simulink model "AC_Feeder"  (R2016b)
settings: Solver=ode1  StartTime=0.0  StopTime=Tsim  FixedStep=Ts  MaxStep=Tsw/20  RelTol=1e-4  EnableMultiTasking=on
values from neighbouring files (symbols this model uses):
  C = 100e-6    (= 0.0001)    [AC_Feeder_Control_Param.m]    (also in AC_Feeder_Control_Param_02-CORPGYEGTI03-P.m; AC_Feeder_Control_Param_02.m; AC_Feeder_Param.m)
  K_pll = dcgain(Gc_pll/tf([1 -Z_pll],[1 -P_pll 0]))    [AC_Feeder_Control_Param.m]    (also in AC_Feeder_Control_Param_02-CORPGYEGTI03-P.m; AC_Feeder_Control_Param_02.m; AC_Feeder_Param.m; gcpll.m)
  Ll = 10e-3    (= 0.01)    [AC_Feeder_Control_Param.m]    (also in AC_Feeder_Control_Param_02-CORPGYEGTI03-P.m; AC_Feeder_Control_Param_02.m; AC_Feeder_Param.m)
  P_pll = res(2)    [AC_Feeder_Control_Param.m]    (also in AC_Feeder_Control_Param_02-CORPGYEGTI03-P.m; AC_Feeder_Control_Param_02.m; AC_Feeder_Param.m = ans(2); gcpll.m = res(1))
  R = 10    [AC_Feeder_Control_Param.m]    (also in AC_Feeder_Control_Param_02-CORPGYEGTI03-P.m; AC_Feeder_Control_Param_02.m; AC_Feeder_Param.m)
  Rl = 0.1    [AC_Feeder_Control_Param.m]    (also in AC_Feeder_Control_Param_02-CORPGYEGTI03-P.m; AC_Feeder_Control_Param_02.m; AC_Feeder_Param.m)
  Ts = 50e-6    (= 5e-05)    [AC_Feeder_Control_Param.m]    (also in AC_Feeder_Control_Param_02-CORPGYEGTI03-P.m; AC_Feeder_Control_Param_02.m; AC_Feeder_Param.m; Feeder_Param.m = 0.0001)
  Tsim = 1    [AC_Feeder_Control_Param.m]    (also in AC_Feeder_Control_Param_02-CORPGYEGTI03-P.m; AC_Feeder_Control_Param_02.m; AC_Feeder_Param.m)
  VLNpk = VLNrms*sqrt(2)    [AC_Feeder_Control_Param.m]    (also in AC_Feeder_Control_Param_02-CORPGYEGTI03-P.m; AC_Feeder_Control_Param_02.m; AC_Feeder_Param.m = VLLrms*sqrt(2/3))
  w1 = 2*pi*f1    (= 376.991118431)    [AC_Feeder_Control_Param.m]    (also in AC_Feeder_Control_Param_02-CORPGYEGTI03-P.m; AC_Feeder_Control_Param_02.m; AC_Feeder_Param.m)
  Z_pll = zero(Gc_pll)    [AC_Feeder_Control_Param.m]    (also in AC_Feeder_Control_Param_02-CORPGYEGTI03-P.m; AC_Feeder_Control_Param_02.m; AC_Feeder_Param.m; gcpll.m)
undefined symbols (not defined in the file or in its folder): DiscIntNeverNeededParam
libraries: powerlib x22, simulink x2
settings Model: Creator=daniel  LastModifiedBy=sixifo
settings DataIOCC: LimitDataPoints=on  SaveFormat=Array  SignalLoggingSaveFormat=ModelDataLogs
settings OptimizationCC: ExpressionDepthLimit=2147483647  InitFltsAndDblsToZero=on  LifeSpan=inf
settings DebuggingCC: UnderspecifiedInitializationDetection=Classic  MergeDetectMultiDrivingBlocksExec=none  SolverPrmCheckMsg=warning  FcnCallInpInsideContextMsg=warning  UnconnectedInputMsg=none  UnconnectedOutputMsg=none  UnconnectedLineMsg=none  StateNameClashWarn=warning  SFUnexpectedBacktrackingDiag=warning  SFNoUnconditionalDefaultTransitionDiag=warning  SFExecutionAtInitializationDiag=none
settings HardwareCC: ProdBitPerPointer=32  ProdBitPerSizeT=32  ProdBitPerPtrDiffT=32  ProdLargestAtomicFloat=None  ProdIntDivRoundTo=Undefined  ProdEndianess=Unspecified  ProdWordSize=32  ProdHWDeviceType=32-bit Generic
settings ModelReferenceCC: PropagateSignalLabelsOutOfModel=off
settings GRTTargetCC: TargetLangStandard=C89/C90 (ANSI)  CombineOutputUpdateFcns=off  GRTInterface=on
settings ConfigComp: CovMetricSettings=dw  CovHtmlReporting=on  CovSaveCumulativeToWorkspaceVar=on  CovSaveSingleToWorkspaceVar=on  CovExternalEMLEnable=off

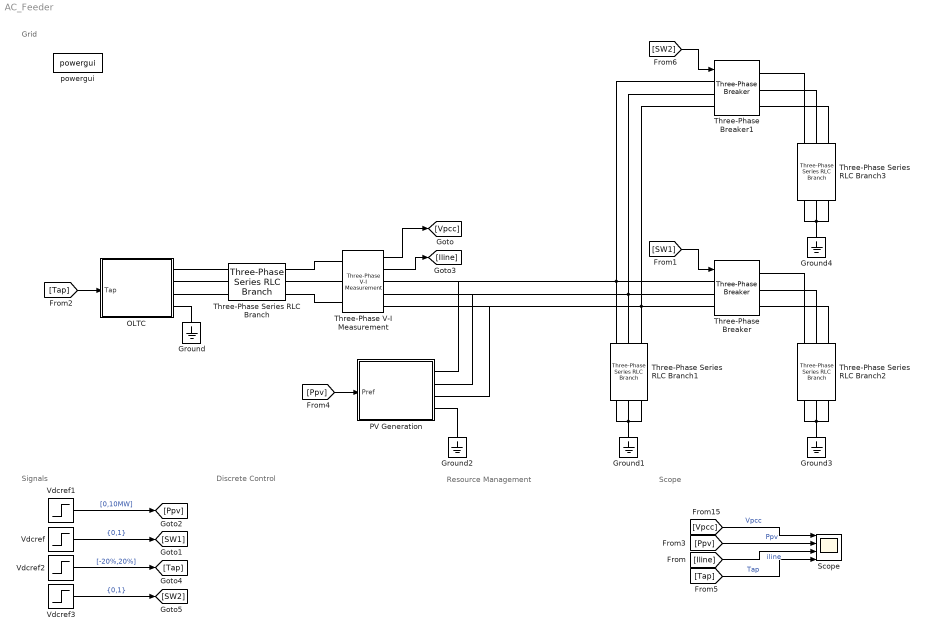
== system AC_Feeder ==
  note: Resource Management
  note: Signals
  note: Discrete Control
  note: Scope
  note: Grid
  Ground{,1..4} (5 alike) : powerlib/Elements/Ground  LConnTagsString=a
  OLTC : Subsystem
  PV Generation : Subsystem
  Scope : Scope  NumInputPorts=4
  Three-Phase Series RLC Branch : powerlib/Elements/Three-Phase Series RLC Branch  LConnTagsString=A|B|C  RConnTagsString=A|B|C  BranchType=RL  Resistance=Rl  Inductance=Ll  Capacitance=1e-6  Measurements=None
  Three-Phase Series RLC Branch1 : powerlib/Elements/Three-Phase Series RLC Branch  LConnTagsString=A|B|C  RConnTagsString=A|B|C  BranchType=R  Resistance=R  Inductance=Ll  Capacitance=1e-6  Measurements=None
  Three-Phase Series RLC Branch2 : powerlib/Elements/Three-Phase Series RLC Branch  LConnTagsString=A|B|C  RConnTagsString=A|B|C  BranchType=R  Resistance=R  Inductance=Ll  Capacitance=1e-6  Measurements=None
  Three-Phase Series RLC Branch3 : powerlib/Elements/Three-Phase Series RLC Branch  LConnTagsString=A|B|C  RConnTagsString=A|B|C  BranchType=C  Resistance=R  Inductance=Ll  Capacitance=C  Measurements=None
  Three-Phase V-I Measurement : powerlib/Measurements/Three-Phase V-I Measurement  VoltageMeasurement=phase-to-ground  SetLabelV=off  LabelV=Vabc  Vpu=off  VpuLL=off  CurrentMeasurement=yes  SetLabelI=off  LabelI=Iabc  Ipu=off  Pbase=100e6  Vbase=500e3  OutputType=Complex  PhasorSimulation=off  PSBequivalent=0
  Three-Phase Breaker : powerlib/Elements/Three-Phase Breaker  InitialState=open  SwitchA=on  SwitchB=on  SwitchC=on  SwitchTimes="[1/60  5/60]"  External=on  BreakerResistance=Ron  SnubberResistance=Rsnubber  SnubberCapacitance=inf  Measurements=None
  Three-Phase Breaker1 : powerlib/Elements/Three-Phase Breaker  InitialState=open  SwitchA=on  SwitchB=on  SwitchC=on  SwitchTimes="[1/60  5/60]"  External=on  BreakerResistance=Ron  SnubberResistance=Rsnubber  SnubberCapacitance=inf  Measurements=None
  Vdcref : Step  Time=Tsim*0.4  SampleTime=0
  Vdcref1 : Step  Time=Tsim*0.20  After=10e6  SampleTime=0
  Vdcref2 : Step  Time=Tsim*0.60  After=10  SampleTime=0
  Vdcref3 : Step  Time=Tsim*0.80  SampleTime=0
  powergui : powerlib/powergui  SimulationMode=Discrete  SolverType=Tustin/Backward Euler (TBE)  SampleTime=50e-6  frequency=60  SPID=off  DisableSnubberDevices=off  DisableRonSwitches=off  DisableVfSwitches=off  SwTol=0  DisplayEquations=off  Interpol=off  ExternalGateDelay=off  methode=off  Ts=0  FunctionMessages=off  echomessages=off  HookPort=off  EnableUseOfTLC=off  x0status=blocks  frequencyindice=0  Pbase=100e6  ErrMax=1e-4  Iterations=50  UnitsV=kV  UnitsW=MW  buscounter=0  RestoreLinks=warning  ResistiveCurrentMeasurement=off  Frange=[0:2:500]  Ylog=off  Xlog=on  ShowGrid=off  save=off  variable=ZData  structure=IL  ZoomFFT=off  StartTime=0  cycles=1  DisplayStyle=1  fundamental=1e4  FreqAxis=off  MaxFrequency=10000  frequencyindicesteady=1  RmsSteady=1  display=off
  wires:
  Vdcref/1 -> [SW1]  "{0,1}"
  [Ppv] -> Scope/2  "Ppv"
  [Tap] -> Scope/4  "Tap"
  [Vpcc] -> Scope/1  "Vpcc"
  [Ppv] -> PV Generation/1(Pref)
  [Iline] -> Scope/3  "iline"
  Vdcref1/1 -> [Ppv]  "[0,10MW]"
  [SW1] -> Three-Phase Breaker/1
  Three-Phase V-I Measurement/1 -> [Vpcc]
  Three-Phase V-I Measurement/2 -> [Iline]
  Vdcref2/1 -> [Tap]  "[-20%,20%]"
  [Tap] -> OLTC/1(Tap)
  Vdcref3/1 -> [SW2]  "{0,1}"
  [SW2] -> Three-Phase Breaker1/1
  connections:
  Ground1/LConn1 -- Three-Phase Series RLC Branch1/RConn3 -- Three-Phase Series RLC Branch1/RConn1 -- Three-Phase Series RLC Branch1/RConn2
  OLTC/RConn1 -- Three-Phase Series RLC Branch/LConn1
  OLTC/RConn2 -- Three-Phase Series RLC Branch/LConn2
  OLTC/RConn3 -- Three-Phase Series RLC Branch/LConn3
  Three-Phase V-I Measurement/RConn1 -- PV Generation/RConn1 -- Three-Phase Breaker1/LConn1 -- Three-Phase Breaker/LConn1 -- Three-Phase Series RLC Branch1/LConn1
  Three-Phase V-I Measurement/RConn2 -- PV Generation/RConn2 -- Three-Phase Breaker1/LConn2 -- Three-Phase Breaker/LConn2 -- Three-Phase Series RLC Branch1/LConn2
  Three-Phase V-I Measurement/RConn3 -- PV Generation/RConn3 -- Three-Phase Breaker1/LConn3 -- Three-Phase Breaker/LConn3 -- Three-Phase Series RLC Branch1/LConn3
  PV Generation/RConn4 -- Ground2/LConn1
  Ground3/LConn1 -- Three-Phase Series RLC Branch2/RConn3 -- Three-Phase Series RLC Branch2/RConn1 -- Three-Phase Series RLC Branch2/RConn2
  Three-Phase Breaker/RConn3 -- Three-Phase Series RLC Branch2/LConn3
  Three-Phase Breaker/RConn2 -- Three-Phase Series RLC Branch2/LConn2
  Three-Phase Breaker/RConn1 -- Three-Phase Series RLC Branch2/LConn1
  Three-Phase Series RLC Branch/RConn2 -- Three-Phase V-I Measurement/LConn2
  Three-Phase Series RLC Branch/RConn1 -- Three-Phase V-I Measurement/LConn1
  Three-Phase Series RLC Branch/RConn3 -- Three-Phase V-I Measurement/LConn3
  OLTC/RConn4 -- Ground/LConn1
  Ground4/LConn1 -- Three-Phase Series RLC Branch3/RConn3 -- Three-Phase Series RLC Branch3/RConn1 -- Three-Phase Series RLC Branch3/RConn2
  Three-Phase Series RLC Branch3/LConn2 -- Three-Phase Breaker1/RConn2
  Three-Phase Breaker1/RConn3 -- Three-Phase Series RLC Branch3/LConn3
  Three-Phase Breaker1/RConn1 -- Three-Phase Series RLC Branch3/LConn1

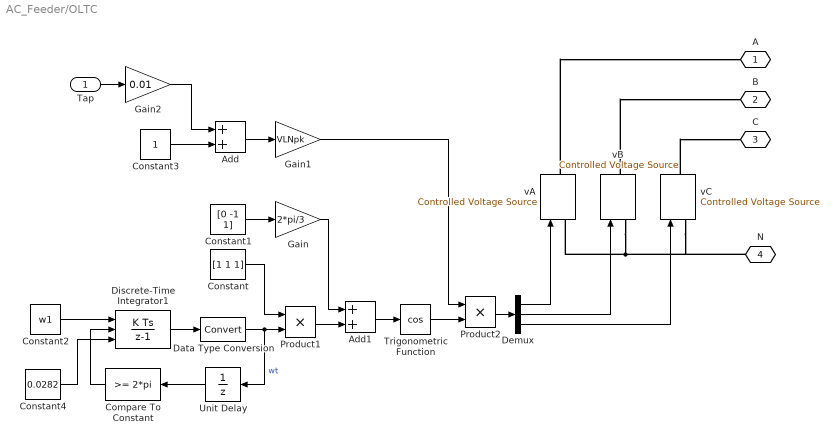
== system AC_Feeder/OLTC ==
  Tap : Inport
  Add : Sum
  Add1 : Sum
  Compare To Constant : simulink/Logic and Bit Operations/Compare To Constant  relop=>=  const=2*pi  OutDataTypeStr=boolean
  Constant : Constant  Value=[1 1 1]
  Constant1 : Constant  Value=[0 -1 1]
  Constant2 : Constant  Value=w1
  Constant3 : Constant
  Constant4 : Constant  Value=0.0282
  Data Type Conversion : DataTypeConversion
  Demux : Demux  Outputs=3
  Discrete-Time Integrator1 : DiscreteIntegrator  gainval=1  ExternalReset=rising  InitialConditionSource=external  SampleTime=Ts  UpperSaturationLimit=0.5*pi  LowerSaturationLimit=0.0001  ICPrevOutput=DiscIntNeverNeededParam  ICPrevScaledInput=DiscIntNeverNeededParam
  Gain : Gain  Gain=2*pi/3
  Gain1 : Gain  Gain=VLNpk
  Gain2 : Gain  Gain=0.01
  Product1 : Product
  Product2 : Product
  Trigonometric Function : Trigonometry  Operator=cos
  Unit Delay : UnitDelay  SampleTime=-1
  vA : powerlib/Electrical Sources/Controlled Voltage Source  Initialize=on  Source_Type=AC  Amplitude=0  Phase=0  Frequency=0  Measurements=None
  vB : powerlib/Electrical Sources/Controlled Voltage Source  Initialize=on  Source_Type=AC  Amplitude=0  Phase=0  Frequency=0  Measurements=None
  vC : powerlib/Electrical Sources/Controlled Voltage Source  Initialize=on  Source_Type=AC  Amplitude=0  Phase=0  Frequency=0  Measurements=None
  A : PMIOPort  Port=1  Side=Right
  B : PMIOPort  Port=2  Side=Right
  C : PMIOPort  Port=3  Side=Right
  N : PMIOPort  Port=4  Side=Right
  wires:
  Demux/1 -> vA/1
  Demux/2 -> vB/1
  Demux/3 -> vC/1
  Product1/1 -> Add1/2
  Constant1/1 -> Gain/1
  Add1/1 -> Trigonometric Function/1
  Constant/1 -> Product1/1
  Gain/1 -> Add1/1
  Trigonometric Function/1 -> Product2/2
  Product2/1 -> Demux/1
  Add/1 -> Gain1/1
  Constant3/1 -> Add/2
  Gain1/1 -> Product2/1
  Gain2/1 -> Add/1
  Tap/1 -> Gain2/1
  Data Type Conversion/1 -> Unit Delay/1, Product1/2  "wt"
  Unit Delay/1 -> Compare To Constant/1
  Discrete-Time Integrator1/1 -> Data Type Conversion/1
  Compare To Constant/1 -> Discrete-Time Integrator1/2
  Constant4/1 -> Discrete-Time Integrator1/3
  Constant2/1 -> Discrete-Time Integrator1/1
  connections:
  vB/LConn1 -- N/RConn1 -- vC/LConn1 -- vA/LConn1
  vA/RConn1 -- A/RConn1
  vB/RConn1 -- B/RConn1
  vC/RConn1 -- C/RConn1

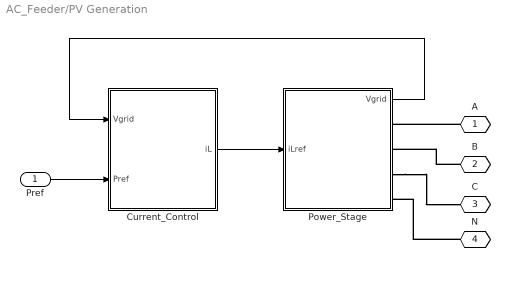
== system AC_Feeder/PV Generation ==
  Pref : Inport
  Current_Control : Subsystem
  Power_Stage : Subsystem
  A : PMIOPort  Port=1  Side=Right
  B : PMIOPort  Port=2  Side=Right
  C : PMIOPort  Port=3  Side=Right
  N : PMIOPort  Port=4  Side=Right
  wires:
  Pref/1 -> Current_Control/2(Pref)
  Power_Stage/1(Vgrid) -> Current_Control/1(Vgrid)
  Current_Control/1(iL) -> Power_Stage/1(iLref)
  connections:
  A/RConn1 -- Power_Stage/RConn1
  B/RConn1 -- Power_Stage/RConn2
  Power_Stage/RConn3 -- C/RConn1
  N/RConn1 -- Power_Stage/RConn4

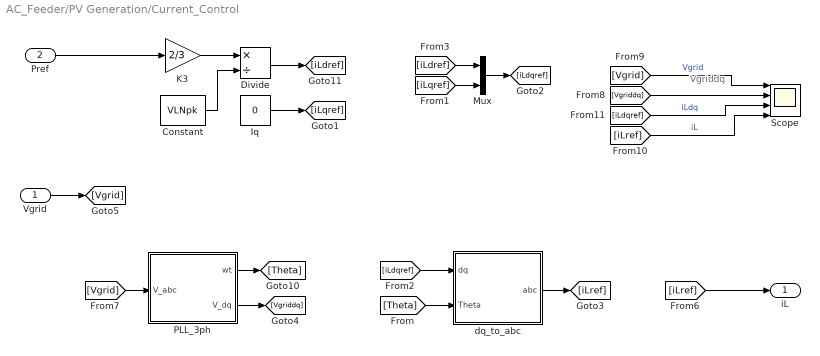
== system AC_Feeder/PV Generation/Current_Control ==
  note: Vgriddq
  Vgrid : Inport
  Pref : Inport  Port=2
  Constant : Constant  Value=VLNpk
  Divide : Product  Inputs=*/
  Iq : Constant  Value=0
  K3 : Gain  Gain=2/3
  Mux : Mux  Inputs=2
  PLL_3ph : Subsystem
  Scope : Scope  NumInputPorts=4
  dq_to_abc : Subsystem
  iL : Outport
  wires:
  [iLdref] -> Mux/1
  K3/1 -> Divide/1
  Pref/1 -> K3/1
  Constant/1 -> Divide/2
  Divide/1 -> [iLdref]
  [iLqref] -> Mux/2
  [Vgrid] -> PLL_3ph/1(V_abc)
  PLL_3ph/2(V_dq) -> [Vgriddq]
  PLL_3ph/1(wt) -> [Theta]
  Vgrid/1 -> [Vgrid]
  Iq/1 -> [iLqref]
  Mux/1 -> [iLdqref]
  [Theta] -> dq_to_abc/2(Theta)
  [iLdqref] -> dq_to_abc/1(dq)
  dq_to_abc/1(abc) -> [iLref]
  [iLref] -> iL/1
  [Vgriddq] -> Scope/2
  [Vgrid] -> Scope/1  "Vgrid"
  [iLdqref] -> Scope/3  "iLdq"
  [iLref] -> Scope/4  "iL"

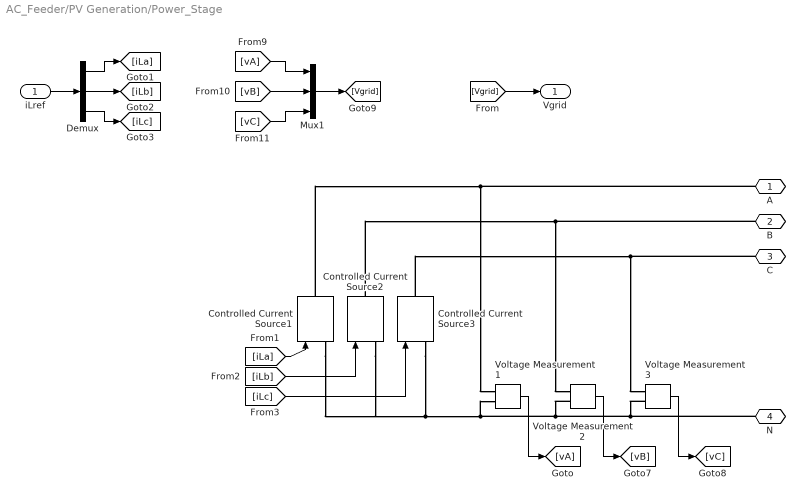
== system AC_Feeder/PV Generation/Power_Stage ==
  iLref : Inport
  Controlled Current Source1 : powerlib/Electrical Sources/Controlled Current Source  Initialize=on  Source_Type=AC  Amplitude=0  Phase=0  Frequency=0  Measurements=None
  Controlled Current Source2 : powerlib/Electrical Sources/Controlled Current Source  Initialize=on  Source_Type=AC  Amplitude=0  Phase=0  Frequency=0  Measurements=None
  Controlled Current Source3 : powerlib/Electrical Sources/Controlled Current Source  Initialize=on  Source_Type=AC  Amplitude=0  Phase=0  Frequency=0  Measurements=None
  Demux : Demux  Outputs=3
  Mux1 : Mux  Inputs=3
  Voltage Measurement 1 : powerlib/Measurements/Voltage Measurement  PhasorSimulation=off  OutputType=Complex  PSBequivalent=0
  Voltage Measurement 2 : powerlib/Measurements/Voltage Measurement  PhasorSimulation=off  OutputType=Complex  PSBequivalent=0
  Voltage Measurement 3 : powerlib/Measurements/Voltage Measurement  PhasorSimulation=off  OutputType=Complex  PSBequivalent=0
  A : PMIOPort  Port=1  Side=Right
  B : PMIOPort  Port=2  Side=Right
  C : PMIOPort  Port=3  Side=Right
  N : PMIOPort  Port=4  Side=Right
  Vgrid : Outport
  wires:
  Voltage Measurement 3/1 -> [vC]
  Voltage Measurement 2/1 -> [vB]
  Voltage Measurement 1/1 -> [vA]
  Mux1/1 -> [Vgrid]
  [vC] -> Mux1/3
  [vA] -> Mux1/1
  [vB] -> Mux1/2
  [Vgrid] -> Vgrid/1
  iLref/1 -> Demux/1
  Demux/1 -> [iLa]
  Demux/2 -> [iLb]
  Demux/3 -> [iLc]
  [iLa] -> Controlled Current Source1/1
  [iLb] -> Controlled Current Source2/1
  [iLc] -> Controlled Current Source3/1
  connections:
  Voltage Measurement 3/LConn2 -- N/RConn1 -- Controlled Current Source1/LConn1 -- Controlled Current Source2/LConn1 -- Controlled Current Source3/LConn1 -- Voltage Measurement 1/LConn2 -- Voltage Measurement 2/LConn2
  C/RConn1 -- Controlled Current Source3/RConn1 -- Voltage Measurement 3/LConn1
  B/RConn1 -- Controlled Current Source2/RConn1 -- Voltage Measurement 2/LConn1
  A/RConn1 -- Controlled Current Source1/RConn1 -- Voltage Measurement 1/LConn1

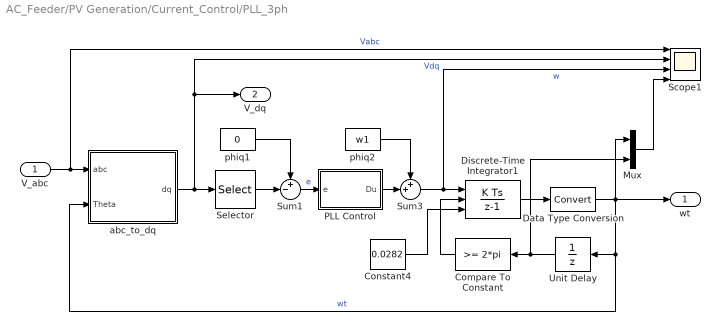
== system AC_Feeder/PV Generation/Current_Control/PLL_3ph ==
  V_abc : Inport
  Compare To Constant : simulink/Logic and Bit Operations/Compare To Constant  relop=>=  const=2*pi  OutDataTypeStr=boolean
  Constant4 : Constant  Value=0.0282
  Data Type Conversion : DataTypeConversion
  Discrete-Time Integrator1 : DiscreteIntegrator  gainval=1  ExternalReset=rising  InitialConditionSource=external  SampleTime=Ts  UpperSaturationLimit=0.5*pi  LowerSaturationLimit=0.0001  ICPrevOutput=DiscIntNeverNeededParam  ICPrevScaledInput=DiscIntNeverNeededParam
  Mux : Mux  Inputs=2
  PLL Control : Subsystem
  Scope1 : Scope  NumInputPorts=4
  Selector : Selector  InputPortWidth=2  IndexOptions=Index vector (dialog)  Indices=[2]  OutputSizes=1
  Sum1 : Sum  Inputs=+-|  SaturateOnIntegerOverflow=on
  Sum3 : Sum  Inputs=++|  SaturateOnIntegerOverflow=on
  Unit Delay : UnitDelay  SampleTime=-1
  abc_to_dq : Subsystem
  phiq1 : Constant  Value=0  OutDataTypeStr=single
  phiq2 : Constant  Value=w1  OutDataTypeStr=single
  wt : Outport
  V_dq : Outport  Port=2
  wires:
  Sum3/1 -> Scope1/3, Discrete-Time Integrator1/1  "w"
  phiq2/1 -> Sum3/1
  V_abc/1 -> abc_to_dq/1(abc), Scope1/1  "Vabc"
  Discrete-Time Integrator1/1 -> Data Type Conversion/1
  Compare To Constant/1 -> Discrete-Time Integrator1/2
  Constant4/1 -> Discrete-Time Integrator1/3
  PLL Control/1(Du) -> Sum3/2
  abc_to_dq/1(dq) -> Selector/1, V_dq/1, Scope1/2  "Vdq"
  Sum1/1 -> PLL Control/1(e)  "e"
  phiq1/1 -> Sum1/1
  Selector/1 -> Sum1/2
  Data Type Conversion/1 -> Mux/1, Unit Delay/1, abc_to_dq/2(Theta), wt/1  "wt"
  Unit Delay/1 -> Mux/2, Compare To Constant/1
  Mux/1 -> Scope1/4

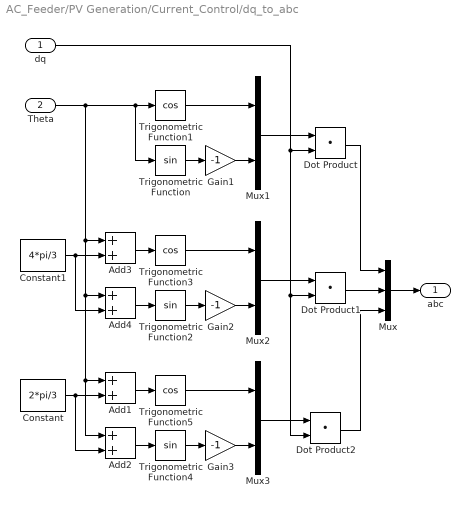
== system AC_Feeder/PV Generation/Current_Control/dq_to_abc ==
  dq : Inport
  Theta : Inport  Port=2
  Add{1..4} (4 alike) : Sum
  Constant : Constant  Value=2*pi/3
  Constant1 : Constant  Value=4*pi/3
  Dot Product : DotProduct  InputSameDT=on  OutDataTypeStr=Inherit: Inherit via internal rule
  Dot Product1 : DotProduct  InputSameDT=on  OutDataTypeStr=Inherit: Inherit via internal rule
  Dot Product2 : DotProduct  InputSameDT=on  OutDataTypeStr=Inherit: Inherit via internal rule
  Gain1 : Gain  Gain=-1
  Gain2 : Gain  Gain=-1
  Gain3 : Gain  Gain=-1
  Mux : Mux  Inputs=3
  Mux1 : Mux  Inputs=2
  Mux2 : Mux  Inputs=2
  Mux3 : Mux  Inputs=2
  Trigonometric Function : Trigonometry
  Trigonometric Function1 : Trigonometry  Operator=cos
  Trigonometric Function2 : Trigonometry
  Trigonometric Function3 : Trigonometry  Operator=cos
  Trigonometric Function4 : Trigonometry
  Trigonometric Function5 : Trigonometry  Operator=cos
  abc : Outport
  wires:
  dq/1 -> Dot Product/2, Dot Product1/2, Dot Product2/2
  Mux/1 -> abc/1
  Mux1/1 -> Dot Product/1
  Dot Product/1 -> Mux/1
  Dot Product1/1 -> Mux/2
  Gain1/1 -> Mux1/2
  Trigonometric Function/1 -> Gain1/1
  Trigonometric Function1/1 -> Mux1/1
  Theta/1 -> Trigonometric Function1/1, Trigonometric Function/1, Add3/1, Add4/1, Add2/1, Add1/1
  Gain2/1 -> Mux2/2
  Trigonometric Function2/1 -> Gain2/1
  Trigonometric Function3/1 -> Mux2/1
  Add4/1 -> Trigonometric Function2/1
  Add3/1 -> Trigonometric Function3/1
  Constant1/1 -> Add3/2, Add4/2
  Gain3/1 -> Mux3/2
  Trigonometric Function4/1 -> Gain3/1
  Trigonometric Function5/1 -> Mux3/1
  Add2/1 -> Trigonometric Function4/1
  Add1/1 -> Trigonometric Function5/1
  Constant/1 -> Add2/2, Add1/2
  Mux2/1 -> Dot Product1/1
  Mux3/1 -> Dot Product2/1
  Dot Product2/1 -> Mux/3

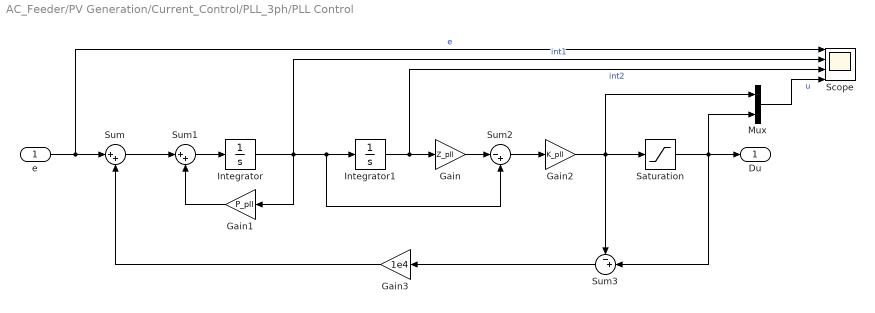
== system AC_Feeder/PV Generation/Current_Control/PLL_3ph/PLL Control ==
  e : Inport
  Gain : Gain  Gain=Z_pll
  Gain1 : Gain  Gain=P_pll
  Gain2 : Gain  Gain=K_pll
  Gain3 : Gain  Gain=1e4
  Integrator : Integrator
  Integrator1 : Integrator
  Mux : Mux  Inputs=2
  Saturation : Saturate  UpperLimit=2*w1  LowerLimit=-2*w1
  Scope : Scope  NumInputPorts=4
  Sum : Sum  Inputs=|++
  Sum1 : Sum  Inputs=|++
  Sum2 : Sum  Inputs=|-+
  Sum3 : Sum  Inputs=-+|
  Du : Outport
  wires:
  Mux/1 -> Scope/4  "u"
  Gain2/1 -> Saturation/1, Sum3/1, Mux/1
  Gain3/1 -> Sum/2
  Sum3/1 -> Gain3/1
  Gain/1 -> Sum2/1
  Sum2/1 -> Gain2/1
  Saturation/1 -> Du/1, Mux/2, Sum3/2
  Integrator1/1 -> Gain/1, Scope/3  "int2"
  Integrator/1 -> Integrator1/1, Sum2/2, Gain1/1, Scope/2  "int1"
  Gain1/1 -> Sum1/2
  Sum1/1 -> Integrator/1
  Sum/1 -> Sum1/1
  e/1 -> Sum/1, Scope/1  "e"

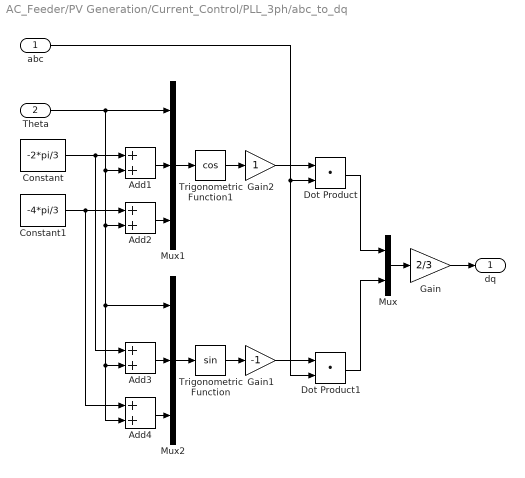
== system AC_Feeder/PV Generation/Current_Control/PLL_3ph/abc_to_dq ==
  abc : Inport
  Theta : Inport  Port=2
  Add{1..4} (4 alike) : Sum
  Constant : Constant  Value=-2*pi/3
  Constant1 : Constant  Value=-4*pi/3
  Dot Product : DotProduct  InputSameDT=on  OutDataTypeStr=Inherit: Inherit via internal rule
  Dot Product1 : DotProduct  InputSameDT=on  OutDataTypeStr=Inherit: Inherit via internal rule
  Gain : Gain  Gain=2/3
  Gain1 : Gain  Gain=-1
  Gain2 : Gain
  Mux : Mux  Inputs=2
  Mux1 : Mux  Inputs=3
  Mux2 : Mux  Inputs=3
  Trigonometric Function : Trigonometry
  Trigonometric Function1 : Trigonometry  Operator=cos
  dq : Outport
  wires:
  Dot Product1/1 -> Mux/2
  Dot Product/1 -> Mux/1
  Gain1/1 -> Dot Product1/1
  Trigonometric Function/1 -> Gain1/1
  Trigonometric Function1/1 -> Gain2/1
  Mux2/1 -> Trigonometric Function/1
  Add4/1 -> Mux2/3
  Add3/1 -> Mux2/2
  Mux1/1 -> Trigonometric Function1/1
  Add2/1 -> Mux1/3
  Constant1/1 -> Add4/1, Add2/1
  Add1/1 -> Mux1/2
  Theta/1 -> Mux1/1, Add3/2, Add4/2, Mux2/1, Add2/2, Add1/2
  Constant/1 -> Add1/1, Add3/1
  Gain/1 -> dq/1
  Mux/1 -> Gain/1
  abc/1 -> Dot Product1/2, Dot Product/2
  Gain2/1 -> Dot Product/1
